simulink model "smoothangle"  (Simulink 6.0)
settings: Solver=ode45  StartTime=0.0  StopTime=10.0  RelTol=1e-3
settings Model: Creator=arnav  LastModifiedBy=batserve  ExtModeAutoUpdateStatusClock=off
settings OptimizationCC: BooleanDataType=off
settings DebuggingCC: SolverPrmCheckMsg=none
settings HardwareCC: TargetUnknown=on

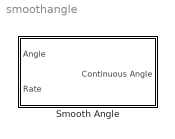
== system smoothangle ==
  Smooth Angle : Subsystem  mask{rad=rad, rads=rad/s}
      mask prompts: rad "Angle measured in:"; rads "Rate measured in:"
      mask help: Constructs continuous angle from angular velocity rate and piecewise continuous angle measured by Joint Sensor on a revolute primitive. Integrates angular velocity to determine number of revolutions that the joint primitive has undergone.
      mask StyleString: popup(rad|deg),popup(rad/s|deg/s)

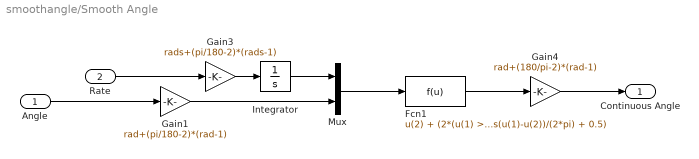
== system smoothangle/Smooth Angle ==
  Angle : Inport  Port=1  LatchInput=off
  Rate : Inport  Port=2  LatchInput=off
  Fcn1 : Fcn  Expr=u(2) + (2*(u(1) > u(2)) - 1)*2*pi*floor(abs(u(1)-u(2))/(2*pi) + 0.5)
  Gain1 : Gain  Gain=rad+(pi/180-2)*(rad-1)  SaturateOnIntegerOverflow=on
  Gain3 : Gain  Gain=rads+(pi/180-2)*(rads-1)  SaturateOnIntegerOverflow=on
  Gain4 : Gain  Gain=rad+(180/pi-2)*(rad-1)  SaturateOnIntegerOverflow=on
  Integrator : Integrator  AbsoluteTolerance=1e-3
  Mux : Mux  Inputs=2
  Continuous Angle : Outport
  wires:
  Angle/1 -> Gain1/1
  Rate/1 -> Gain3/1
  Fcn1/1 -> Gain4/1
  Mux/1 -> Fcn1/1
  Integrator/1 -> Mux/1
  Gain3/1 -> Integrator/1
  Gain1/1 -> Mux/2
  Gain4/1 -> Continuous Angle/1
